simulink model "DPL1"  (R2016a)
settings: Solver=ode23tb  StartTime=0.0  StopTime=0.05  MaxStep=1e-4  RelTol=1e-5
libraries: powerlib x9
settings Model: Creator=dutch  LastModifiedBy=dutch

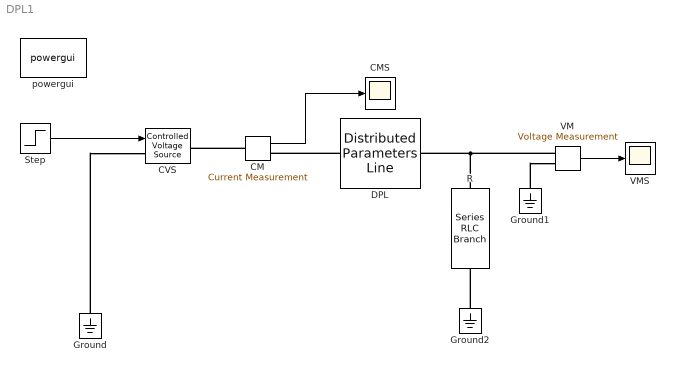
== system DPL1 ==
  CM : powerlib/Measurements/Current Measurement  PhasorSimulation=off  OutputType=Complex  PSBequivalent=0
  CMS : Scope
  CVS : powerlib/Electrical Sources/Controlled Voltage Source  Initialize=off  Source_Type=DC  Amplitude=0  Phase=0  Frequency=0  Measurements=None
  DPL : powerlib/Elements/Distributed Parameters Line  Phases=1  Frequency=50  Resistance=0  Inductance=5e-4  Capacitance=50e-9  Length=1000  x1=[0;0;1.5707963267949]  x2=[0;0;1.5707963267949]  x3=[0;0;1.5707963267949]  x4=[0;0;1.5707963267949]  x5=0.005  V1=[0;0;1.571]  V2=[0;0;1.571]  I1=[0;0;1.571]  I2=[0;0;1.571]  nHarmo=1  Measurements=None
  Ground : powerlib/Elements/Ground  LConnTagsString=a
  Ground1 : powerlib/Elements/Ground  LConnTagsString=a
  Ground2 : powerlib/Elements/Ground  LConnTagsString=a
  R : powerlib/Elements/Series RLC Branch  LConnTagsString=__new0  RConnTagsString=__new0  BranchType=R  Resistance=inf  Inductance=1e-3  SetiL0=off  InitialCurrent=0  Capacitance=1e-6  Setx0=off  InitialVoltage=0  Measurements=None
  Step : Step  Time=0  After=10  SampleTime=0
  VM : powerlib/Measurements/Voltage Measurement  PhasorSimulation=off  OutputType=Complex  PSBequivalent=0
  VMS : Scope
  powergui : powerlib/powergui  Priority=1  SimulationMode=Continuous  SolverType=Tustin/Backward Euler (TBE)  SampleTime=50e-6  frequency=60  SPID=on  DisableSnubberDevices=off  DisableRonSwitches=off  DisableVfSwitches=off  SwTol=0  DisplayEquations=off  Interpol=off  ExternalGateDelay=off  methode=off  Ts=10  FunctionMessages=off  echomessages=off  HookPort=off  EnableUseOfTLC=off  x0status=blocks  frequencyindice=0  Pbase=100e6  ErrMax=1e-4  Iterations=50  UnitsV=kV  UnitsW=MW  buscounter=0  RestoreLinks=warning  ResistiveCurrentMeasurement=off  Frange=[0:2:500]  Ylog=off  Xlog=on  ShowGrid=off  save=off  variable=ZData  structure=0  ZoomFFT=off  StartTime=0.0  cycles=1  DisplayStyle=1  fundamental=60  FreqAxis=off  MaxFrequency=1000  frequencyindicesteady=1  RmsSteady=1  display=off
  wires:
  CM/1 -> CMS/1
  VM/1 -> VMS/1
  Step/1 -> CVS/1
  connections:
  Ground/LConn1 -- CVS/LConn1
  VM/LConn1 -- DPL/RConn1 -- R/LConn1
  CM/LConn1 -- CVS/RConn1
  DPL/LConn1 -- CM/RConn1
  Ground1/LConn1 -- VM/LConn2
  Ground2/LConn1 -- R/RConn1
